simulink model "Test_FourMotor_PID_simcape_motor"  (R2025a)
settings: Solver=FixedStepAuto  StartTime=0.0  StopTime=2  FixedStep=50e-5  RelTol=1e-3
values from neighbouring files (symbols this model uses):
  Ki_id = 710.3004    [EMRAX348_DQData.m]    (also in Evolito_D500_DQData.m = 281.669634183)
  Ki_iq = 1.0615e3    (= 1061.5)    [EMRAX348_DQData.m]    (also in Evolito_D500_DQData.m = 420.937840785)
  Kp_id = 0.8779    [EMRAX348_DQData.m]    (also in Evolito_D500_DQData.m = 0.144107025607)
  Kp_iq = 1.0744    [EMRAX348_DQData.m]    (also in Evolito_D500_DQData.m = 0.144418307682)
  Ld = 52e-6    (= 5.2e-05)    [EMRAX348_DQData.m]    (also in Evolito_D500_DQData.m = 4e-05; pmsm_batt_testbench_data.m = 4e-05)
  Lq = 52e-6    (= 5.2e-05)    [EMRAX348_DQData.m]    (also in Evolito_D500_DQData.m = 4e-05; pmsm_batt_testbench_data.m = 4e-05)
  p = 10    [EMRAX348_DQData.m]    (also in Evolito_D500_DQData.m; pmsm_batt_testbench_data.m)
  psim = 0.06249    [EMRAX348_DQData.m]    (also in Evolito_D500_DQData.m = 0.045; pmsm_batt_testbench_data.m = 0.045)
undefined symbols (not defined in the file or in its folder): Limit, motorctrl, RPM
libraries: fl_lib x101, nesl_utility x37, eeDiscretePi x8, slpidlib x7, eeDqVoltageLimiter x4, eePmsmCurrentReferenceGen x4, eePmsmTorqueEstimator x4, ee_lib x4, batteryecm_lib x2, HEV_Battery_Lib x1, spspowerguiLib x1
(part 3 of 3)

== system Test_FourMotor_PID_simcape_motor/Detailed/Electric Drive/Sensor ==
  Filter A : TransferFcn  Denominator=[1e-4 1]
  Filter w : TransferFcn  Denominator=[1e-4 1]
  MRRef : fl_lib/Mechanical/Rotational Elements/Mechanical Rotational Reference
  Motion Sensor : fl_lib/Mechanical/Mechanical Sensors/Ideal Rotational Motion Sensor  reference=foundation.enum.MeasurementReference.difference  acceleration_port=false  velocity_port=true  position_port=true  wrap_angle=simscape.enum.onoff.off  offset=0 deg
  PS-Simulink Converter1 : nesl_utility/PS-Simulink Converter  PhysicalDomain=network_engine_domain  SubClassName=ps_output  LeftPortType=input  RightPortType=output  PseudoPeriodic=off  Frequencies=[]  VectorFormat=1-D array  Unit=rad/s  AffineConversion=off
  PS-Simulink Converter2 : nesl_utility/PS-Simulink Converter  PhysicalDomain=network_engine_domain  SubClassName=ps_output  LeftPortType=input  RightPortType=output  PseudoPeriodic=off  Frequencies=[]  VectorFormat=1-D array  Unit=rad  AffineConversion=off
  R : PMIOPort  Side=Left
  C : PMIOPort  Port=2  Side=Right
  w : Outport  VectorParamsAs1DForOutWhenUnconnected=off
  A : Outport  Port=2  VectorParamsAs1DForOutWhenUnconnected=off
  wires:
  PS-Simulink Converter1/1 -> Filter w/1
  PS-Simulink Converter2/1 -> Filter A/1
  Filter A/1 -> A/1
  Filter w/1 -> w/1
  connections:
  Motion Sensor/RConn2 -- PS-Simulink Converter1/LConn1
  Motion Sensor/RConn1 -- MRRef/LConn1
  C/RConn1 -- R/RConn1 -- Motion Sensor/LConn1
  Motion Sensor/RConn3 -- PS-Simulink Converter2/LConn1

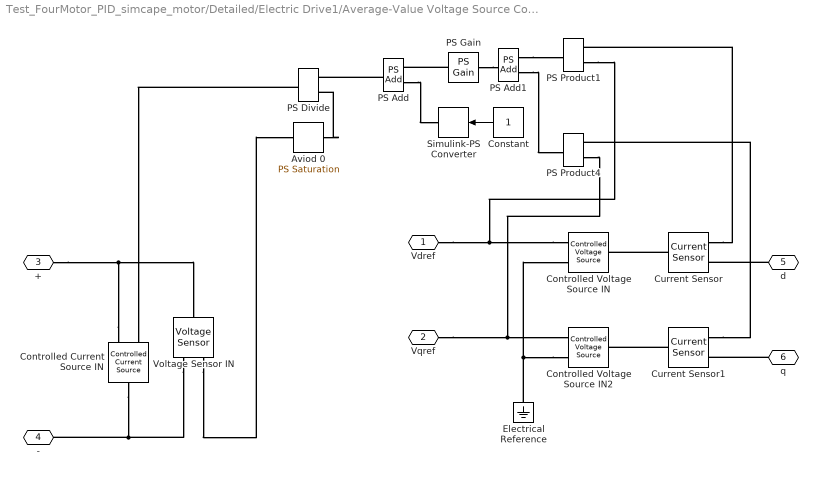
== system Test_FourMotor_PID_simcape_motor/Detailed/Electric Drive1/Average-Value Voltage Source Converter dq0 ==
  Aviod 0 : fl_lib/Physical Signals/Nonlinear Operators/PS Saturation  upper_limit=inf V  lower_limit=1e-6 V  ZeroCross=true
  Constant : Constant  SampleTime=0
  Controlled Current Source IN : fl_lib/Electrical/Electrical Sources/Controlled Current Source
  Controlled Voltage Source IN : fl_lib/Electrical/Electrical Sources/Controlled Voltage Source
  Controlled Voltage Source IN2 : fl_lib/Electrical/Electrical Sources/Controlled Voltage Source
  Current Sensor : fl_lib/Electrical/Electrical Sensors/Current Sensor
  Current Sensor1 : fl_lib/Electrical/Electrical Sensors/Current Sensor
  Electrical Reference : fl_lib/Electrical/Electrical Elements/Electrical Reference
  PS Add : fl_lib/Physical Signals/Functions/PS Add
  PS Add1 : fl_lib/Physical Signals/Functions/PS Add
  PS Divide : fl_lib/Physical Signals/Functions/PS Divide
  PS Gain : fl_lib/Physical Signals/Functions/PS Gain  gain=3/2
  PS Product1 : fl_lib/Physical Signals/Functions/PS Product
  PS Product4 : fl_lib/Physical Signals/Functions/PS Product
  Simulink-PS Converter : nesl_utility/Simulink-PS Converter  PhysicalDomain=network_engine_domain  SubClassName=ps_input  LeftPortType=input  RightPortType=output  PseudoPeriodic=off  Frequencies=[]  NoiseDistribution=none  NoiseParameters=[]  Unit=W  AffineConversion=off  FilteringAndDerivatives=provide  SimscapeFilterOrder=1  InputFilterTimeConstant=0.001  UdotUserProvided=0
  Voltage Sensor IN : fl_lib/Electrical/Electrical Sensors/Voltage Sensor
  Vdref : PMIOPort  Side=Left
  Vqref : PMIOPort  Port=2  Side=Left
  + : PMIOPort  Port=3  Side=Left
  - : PMIOPort  Port=4  Side=Left
  d : PMIOPort  Port=5  Side=Right
  q : PMIOPort  Port=6  Side=Right
  wires:
  Constant/1 -> Simulink-PS Converter/1
  connections:
  Controlled Current Source IN/RConn2 -- Voltage Sensor IN/LConn1 -- +/RConn1
  -/RConn1 -- Voltage Sensor IN/RConn2 -- Controlled Current Source IN/LConn1
  Controlled Voltage Source IN2/RConn2 -- Electrical Reference/LConn1 -- Controlled Voltage Source IN/RConn2
  Current Sensor1/LConn1 -- Controlled Voltage Source IN2/LConn1
  Current Sensor/LConn1 -- Controlled Voltage Source IN/LConn1
  Voltage Sensor IN/RConn1 -- Aviod 0/LConn1
  Controlled Voltage Source IN/RConn1 -- Vdref/RConn1 -- PS Product1/LConn2
  Vqref/RConn1 -- Controlled Voltage Source IN2/RConn1 -- PS Product4/LConn2
  PS Add1/LConn1 -- PS Product1/RConn1
  PS Add1/LConn2 -- PS Product4/RConn1
  Aviod 0/RConn1 -- PS Divide/LConn2
  PS Divide/RConn1 -- Controlled Current Source IN/RConn1
  PS Add/RConn1 -- PS Divide/LConn1
  PS Add/LConn2 -- Simulink-PS Converter/RConn1
  d/RConn1 -- Current Sensor/RConn2
  q/RConn1 -- Current Sensor1/RConn2
  Current Sensor/RConn1 -- PS Product1/LConn1
  Current Sensor1/RConn1 -- PS Product4/LConn1
  PS Gain/LConn1 -- PS Add1/RConn1
  PS Gain/RConn1 -- PS Add/LConn1

== system Test_FourMotor_PID_simcape_motor/Detailed/Electric Drive1/Meas I ==
  Current Sensor d : fl_lib/Electrical/Electrical Sensors/Current Sensor
  Current Sensor q : fl_lib/Electrical/Electrical Sensors/Current Sensor
  Filter id : TransferFcn  Denominator=[1e-4 1]
  Filter iq : TransferFcn  Denominator=[1e-4 1]
  Mux : Mux  Inputs=2
  PS-Simulink Converter : nesl_utility/PS-Simulink Converter  PhysicalDomain=network_engine_domain  SubClassName=ps_output  LeftPortType=input  RightPortType=output  PseudoPeriodic=off  Frequencies=[]  VectorFormat=1-D array  Unit=A  AffineConversion=off
  PS-Simulink Converter1 : nesl_utility/PS-Simulink Converter  PhysicalDomain=network_engine_domain  SubClassName=ps_output  LeftPortType=input  RightPortType=output  PseudoPeriodic=off  Frequencies=[]  VectorFormat=1-D array  Unit=A  AffineConversion=off
  d1 : PMIOPort  Side=Left
  q1 : PMIOPort  Port=2  Side=Left
  d2 : PMIOPort  Port=3  Side=Right
  q2 : PMIOPort  Port=4  Side=Right
  idq : Outport  VectorParamsAs1DForOutWhenUnconnected=off
  wires:
  PS-Simulink Converter1/1 -> Filter iq/1
  PS-Simulink Converter/1 -> Filter id/1
  Mux/1 -> idq/1
  Filter id/1 -> Mux/1
  Filter iq/1 -> Mux/2
  connections:
  d1/RConn1 -- Current Sensor d/LConn1
  Current Sensor q/LConn1 -- q1/RConn1
  Current Sensor d/RConn2 -- d2/RConn1
  q2/RConn1 -- Current Sensor q/RConn2
  PS-Simulink Converter/LConn1 -- Current Sensor d/RConn1
  PS-Simulink Converter1/LConn1 -- Current Sensor q/RConn1

== system Test_FourMotor_PID_simcape_motor/Detailed/Electric Drive1/Meas V ==
  PS-Simulink Converter4 : nesl_utility/PS-Simulink Converter  PhysicalDomain=network_engine_domain  SubClassName=ps_output  LeftPortType=input  RightPortType=output  PseudoPeriodic=off  Frequencies=[]  VectorFormat=1-D array  Unit=V  AffineConversion=off
  Voltage Sensor : fl_lib/Electrical/Electrical Sensors/Voltage Sensor
  - : PMIOPort  Side=Right
  + : PMIOPort  Port=2  Side=Left
  Vdc : Outport  VectorParamsAs1DForOutWhenUnconnected=off
  wires:
  PS-Simulink Converter4/1 -> Vdc/1
  connections:
  PS-Simulink Converter4/LConn1 -- Voltage Sensor/RConn1
  Voltage Sensor/LConn1 -- +/RConn1
  Voltage Sensor/RConn2 -- -/RConn1

== system Test_FourMotor_PID_simcape_motor/Detailed/Electric Drive1/Sensor ==
  Filter A : TransferFcn  Denominator=[1e-4 1]
  Filter w : TransferFcn  Denominator=[1e-4 1]
  MRRef : fl_lib/Mechanical/Rotational Elements/Mechanical Rotational Reference
  Motion Sensor : fl_lib/Mechanical/Mechanical Sensors/Ideal Rotational Motion Sensor  reference=foundation.enum.MeasurementReference.difference  acceleration_port=false  velocity_port=true  position_port=true  wrap_angle=simscape.enum.onoff.off  offset=0 deg
  PS-Simulink Converter1 : nesl_utility/PS-Simulink Converter  PhysicalDomain=network_engine_domain  SubClassName=ps_output  LeftPortType=input  RightPortType=output  PseudoPeriodic=off  Frequencies=[]  VectorFormat=1-D array  Unit=rad/s  AffineConversion=off
  PS-Simulink Converter2 : nesl_utility/PS-Simulink Converter  PhysicalDomain=network_engine_domain  SubClassName=ps_output  LeftPortType=input  RightPortType=output  PseudoPeriodic=off  Frequencies=[]  VectorFormat=1-D array  Unit=rad  AffineConversion=off
  R : PMIOPort  Side=Left
  C : PMIOPort  Port=2  Side=Right
  w : Outport  VectorParamsAs1DForOutWhenUnconnected=off
  A : Outport  Port=2  VectorParamsAs1DForOutWhenUnconnected=off
  wires:
  PS-Simulink Converter1/1 -> Filter w/1
  PS-Simulink Converter2/1 -> Filter A/1
  Filter A/1 -> A/1
  Filter w/1 -> w/1
  connections:
  Motion Sensor/RConn2 -- PS-Simulink Converter1/LConn1
  Motion Sensor/RConn1 -- MRRef/LConn1
  C/RConn1 -- R/RConn1 -- Motion Sensor/LConn1
  Motion Sensor/RConn3 -- PS-Simulink Converter2/LConn1

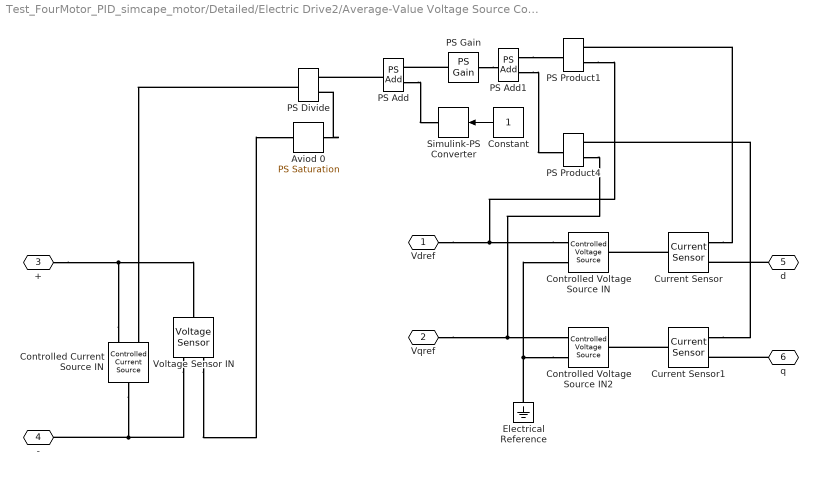
== system Test_FourMotor_PID_simcape_motor/Detailed/Electric Drive2/Average-Value Voltage Source Converter dq0 ==
  Aviod 0 : fl_lib/Physical Signals/Nonlinear Operators/PS Saturation  upper_limit=inf V  lower_limit=1e-6 V  ZeroCross=true
  Constant : Constant  SampleTime=0
  Controlled Current Source IN : fl_lib/Electrical/Electrical Sources/Controlled Current Source
  Controlled Voltage Source IN : fl_lib/Electrical/Electrical Sources/Controlled Voltage Source
  Controlled Voltage Source IN2 : fl_lib/Electrical/Electrical Sources/Controlled Voltage Source
  Current Sensor : fl_lib/Electrical/Electrical Sensors/Current Sensor
  Current Sensor1 : fl_lib/Electrical/Electrical Sensors/Current Sensor
  Electrical Reference : fl_lib/Electrical/Electrical Elements/Electrical Reference
  PS Add : fl_lib/Physical Signals/Functions/PS Add
  PS Add1 : fl_lib/Physical Signals/Functions/PS Add
  PS Divide : fl_lib/Physical Signals/Functions/PS Divide
  PS Gain : fl_lib/Physical Signals/Functions/PS Gain  gain=3/2
  PS Product1 : fl_lib/Physical Signals/Functions/PS Product
  PS Product4 : fl_lib/Physical Signals/Functions/PS Product
  Simulink-PS Converter : nesl_utility/Simulink-PS Converter  PhysicalDomain=network_engine_domain  SubClassName=ps_input  LeftPortType=input  RightPortType=output  PseudoPeriodic=off  Frequencies=[]  NoiseDistribution=none  NoiseParameters=[]  Unit=W  AffineConversion=off  FilteringAndDerivatives=provide  SimscapeFilterOrder=1  InputFilterTimeConstant=0.001  UdotUserProvided=0
  Voltage Sensor IN : fl_lib/Electrical/Electrical Sensors/Voltage Sensor
  Vdref : PMIOPort  Side=Left
  Vqref : PMIOPort  Port=2  Side=Left
  + : PMIOPort  Port=3  Side=Left
  - : PMIOPort  Port=4  Side=Left
  d : PMIOPort  Port=5  Side=Right
  q : PMIOPort  Port=6  Side=Right
  wires:
  Constant/1 -> Simulink-PS Converter/1
  connections:
  Controlled Current Source IN/RConn2 -- Voltage Sensor IN/LConn1 -- +/RConn1
  -/RConn1 -- Voltage Sensor IN/RConn2 -- Controlled Current Source IN/LConn1
  Controlled Voltage Source IN2/RConn2 -- Electrical Reference/LConn1 -- Controlled Voltage Source IN/RConn2
  Current Sensor1/LConn1 -- Controlled Voltage Source IN2/LConn1
  Current Sensor/LConn1 -- Controlled Voltage Source IN/LConn1
  Voltage Sensor IN/RConn1 -- Aviod 0/LConn1
  Controlled Voltage Source IN/RConn1 -- Vdref/RConn1 -- PS Product1/LConn2
  Vqref/RConn1 -- Controlled Voltage Source IN2/RConn1 -- PS Product4/LConn2
  PS Add1/LConn1 -- PS Product1/RConn1
  PS Add1/LConn2 -- PS Product4/RConn1
  Aviod 0/RConn1 -- PS Divide/LConn2
  PS Divide/RConn1 -- Controlled Current Source IN/RConn1
  PS Add/RConn1 -- PS Divide/LConn1
  PS Add/LConn2 -- Simulink-PS Converter/RConn1
  d/RConn1 -- Current Sensor/RConn2
  q/RConn1 -- Current Sensor1/RConn2
  Current Sensor/RConn1 -- PS Product1/LConn1
  Current Sensor1/RConn1 -- PS Product4/LConn1
  PS Gain/LConn1 -- PS Add1/RConn1
  PS Gain/RConn1 -- PS Add/LConn1

== system Test_FourMotor_PID_simcape_motor/Detailed/Electric Drive2/Meas I ==
  Current Sensor d : fl_lib/Electrical/Electrical Sensors/Current Sensor
  Current Sensor q : fl_lib/Electrical/Electrical Sensors/Current Sensor
  Filter id : TransferFcn  Denominator=[1e-4 1]
  Filter iq : TransferFcn  Denominator=[1e-4 1]
  Mux : Mux  Inputs=2
  PS-Simulink Converter : nesl_utility/PS-Simulink Converter  PhysicalDomain=network_engine_domain  SubClassName=ps_output  LeftPortType=input  RightPortType=output  PseudoPeriodic=off  Frequencies=[]  VectorFormat=1-D array  Unit=A  AffineConversion=off
  PS-Simulink Converter1 : nesl_utility/PS-Simulink Converter  PhysicalDomain=network_engine_domain  SubClassName=ps_output  LeftPortType=input  RightPortType=output  PseudoPeriodic=off  Frequencies=[]  VectorFormat=1-D array  Unit=A  AffineConversion=off
  d1 : PMIOPort  Side=Left
  q1 : PMIOPort  Port=2  Side=Left
  d2 : PMIOPort  Port=3  Side=Right
  q2 : PMIOPort  Port=4  Side=Right
  idq : Outport  VectorParamsAs1DForOutWhenUnconnected=off
  wires:
  PS-Simulink Converter1/1 -> Filter iq/1
  PS-Simulink Converter/1 -> Filter id/1
  Mux/1 -> idq/1
  Filter id/1 -> Mux/1
  Filter iq/1 -> Mux/2
  connections:
  d1/RConn1 -- Current Sensor d/LConn1
  Current Sensor q/LConn1 -- q1/RConn1
  Current Sensor d/RConn2 -- d2/RConn1
  q2/RConn1 -- Current Sensor q/RConn2
  PS-Simulink Converter/LConn1 -- Current Sensor d/RConn1
  PS-Simulink Converter1/LConn1 -- Current Sensor q/RConn1

== system Test_FourMotor_PID_simcape_motor/Detailed/Electric Drive2/Meas V ==
  PS-Simulink Converter4 : nesl_utility/PS-Simulink Converter  PhysicalDomain=network_engine_domain  SubClassName=ps_output  LeftPortType=input  RightPortType=output  PseudoPeriodic=off  Frequencies=[]  VectorFormat=1-D array  Unit=V  AffineConversion=off
  Voltage Sensor : fl_lib/Electrical/Electrical Sensors/Voltage Sensor
  - : PMIOPort  Side=Right
  + : PMIOPort  Port=2  Side=Left
  Vdc : Outport  VectorParamsAs1DForOutWhenUnconnected=off
  wires:
  PS-Simulink Converter4/1 -> Vdc/1
  connections:
  PS-Simulink Converter4/LConn1 -- Voltage Sensor/RConn1
  Voltage Sensor/LConn1 -- +/RConn1
  Voltage Sensor/RConn2 -- -/RConn1

== system Test_FourMotor_PID_simcape_motor/Detailed/Electric Drive2/Sensor ==
  Filter A : TransferFcn  Denominator=[1e-4 1]
  Filter w : TransferFcn  Denominator=[1e-4 1]
  MRRef : fl_lib/Mechanical/Rotational Elements/Mechanical Rotational Reference
  Motion Sensor : fl_lib/Mechanical/Mechanical Sensors/Ideal Rotational Motion Sensor  reference=foundation.enum.MeasurementReference.difference  acceleration_port=false  velocity_port=true  position_port=true  wrap_angle=simscape.enum.onoff.off  offset=0 deg
  PS-Simulink Converter1 : nesl_utility/PS-Simulink Converter  PhysicalDomain=network_engine_domain  SubClassName=ps_output  LeftPortType=input  RightPortType=output  PseudoPeriodic=off  Frequencies=[]  VectorFormat=1-D array  Unit=rad/s  AffineConversion=off
  PS-Simulink Converter2 : nesl_utility/PS-Simulink Converter  PhysicalDomain=network_engine_domain  SubClassName=ps_output  LeftPortType=input  RightPortType=output  PseudoPeriodic=off  Frequencies=[]  VectorFormat=1-D array  Unit=rad  AffineConversion=off
  R : PMIOPort  Side=Left
  C : PMIOPort  Port=2  Side=Right
  w : Outport  VectorParamsAs1DForOutWhenUnconnected=off
  A : Outport  Port=2  VectorParamsAs1DForOutWhenUnconnected=off
  wires:
  PS-Simulink Converter1/1 -> Filter w/1
  PS-Simulink Converter2/1 -> Filter A/1
  Filter A/1 -> A/1
  Filter w/1 -> w/1
  connections:
  Motion Sensor/RConn2 -- PS-Simulink Converter1/LConn1
  Motion Sensor/RConn1 -- MRRef/LConn1
  C/RConn1 -- R/RConn1 -- Motion Sensor/LConn1
  Motion Sensor/RConn3 -- PS-Simulink Converter2/LConn1

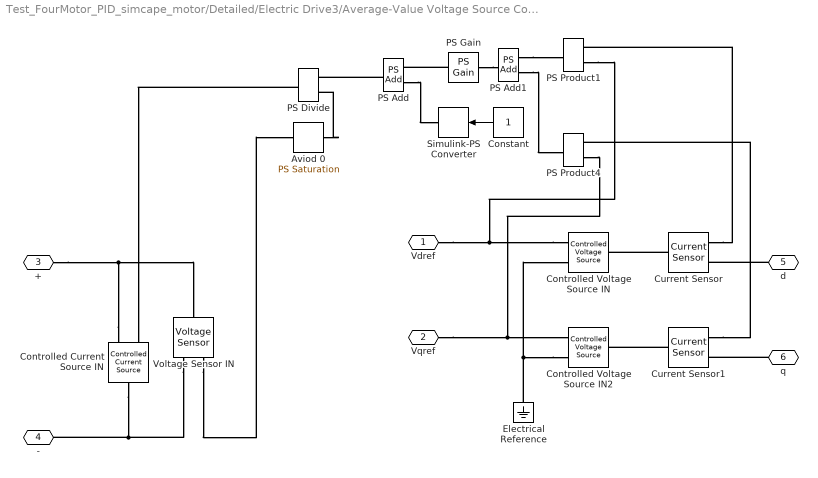
== system Test_FourMotor_PID_simcape_motor/Detailed/Electric Drive3/Average-Value Voltage Source Converter dq0 ==
  Aviod 0 : fl_lib/Physical Signals/Nonlinear Operators/PS Saturation  upper_limit=inf V  lower_limit=1e-6 V  ZeroCross=true
  Constant : Constant  SampleTime=0
  Controlled Current Source IN : fl_lib/Electrical/Electrical Sources/Controlled Current Source
  Controlled Voltage Source IN : fl_lib/Electrical/Electrical Sources/Controlled Voltage Source
  Controlled Voltage Source IN2 : fl_lib/Electrical/Electrical Sources/Controlled Voltage Source
  Current Sensor : fl_lib/Electrical/Electrical Sensors/Current Sensor
  Current Sensor1 : fl_lib/Electrical/Electrical Sensors/Current Sensor
  Electrical Reference : fl_lib/Electrical/Electrical Elements/Electrical Reference
  PS Add : fl_lib/Physical Signals/Functions/PS Add
  PS Add1 : fl_lib/Physical Signals/Functions/PS Add
  PS Divide : fl_lib/Physical Signals/Functions/PS Divide
  PS Gain : fl_lib/Physical Signals/Functions/PS Gain  gain=3/2
  PS Product1 : fl_lib/Physical Signals/Functions/PS Product
  PS Product4 : fl_lib/Physical Signals/Functions/PS Product
  Simulink-PS Converter : nesl_utility/Simulink-PS Converter  PhysicalDomain=network_engine_domain  SubClassName=ps_input  LeftPortType=input  RightPortType=output  PseudoPeriodic=off  Frequencies=[]  NoiseDistribution=none  NoiseParameters=[]  Unit=W  AffineConversion=off  FilteringAndDerivatives=provide  SimscapeFilterOrder=1  InputFilterTimeConstant=0.001  UdotUserProvided=0
  Voltage Sensor IN : fl_lib/Electrical/Electrical Sensors/Voltage Sensor
  Vdref : PMIOPort  Side=Left
  Vqref : PMIOPort  Port=2  Side=Left
  + : PMIOPort  Port=3  Side=Left
  - : PMIOPort  Port=4  Side=Left
  d : PMIOPort  Port=5  Side=Right
  q : PMIOPort  Port=6  Side=Right
  wires:
  Constant/1 -> Simulink-PS Converter/1
  connections:
  Controlled Current Source IN/RConn2 -- Voltage Sensor IN/LConn1 -- +/RConn1
  -/RConn1 -- Voltage Sensor IN/RConn2 -- Controlled Current Source IN/LConn1
  Controlled Voltage Source IN2/RConn2 -- Electrical Reference/LConn1 -- Controlled Voltage Source IN/RConn2
  Current Sensor1/LConn1 -- Controlled Voltage Source IN2/LConn1
  Current Sensor/LConn1 -- Controlled Voltage Source IN/LConn1
  Voltage Sensor IN/RConn1 -- Aviod 0/LConn1
  Controlled Voltage Source IN/RConn1 -- Vdref/RConn1 -- PS Product1/LConn2
  Vqref/RConn1 -- Controlled Voltage Source IN2/RConn1 -- PS Product4/LConn2
  PS Add1/LConn1 -- PS Product1/RConn1
  PS Add1/LConn2 -- PS Product4/RConn1
  Aviod 0/RConn1 -- PS Divide/LConn2
  PS Divide/RConn1 -- Controlled Current Source IN/RConn1
  PS Add/RConn1 -- PS Divide/LConn1
  PS Add/LConn2 -- Simulink-PS Converter/RConn1
  d/RConn1 -- Current Sensor/RConn2
  q/RConn1 -- Current Sensor1/RConn2
  Current Sensor/RConn1 -- PS Product1/LConn1
  Current Sensor1/RConn1 -- PS Product4/LConn1
  PS Gain/LConn1 -- PS Add1/RConn1
  PS Gain/RConn1 -- PS Add/LConn1

== system Test_FourMotor_PID_simcape_motor/Detailed/Electric Drive3/Meas I ==
  Current Sensor d : fl_lib/Electrical/Electrical Sensors/Current Sensor
  Current Sensor q : fl_lib/Electrical/Electrical Sensors/Current Sensor
  Filter id : TransferFcn  Denominator=[1e-4 1]
  Filter iq : TransferFcn  Denominator=[1e-4 1]
  Mux : Mux  Inputs=2
  PS-Simulink Converter : nesl_utility/PS-Simulink Converter  PhysicalDomain=network_engine_domain  SubClassName=ps_output  LeftPortType=input  RightPortType=output  PseudoPeriodic=off  Frequencies=[]  VectorFormat=1-D array  Unit=A  AffineConversion=off
  PS-Simulink Converter1 : nesl_utility/PS-Simulink Converter  PhysicalDomain=network_engine_domain  SubClassName=ps_output  LeftPortType=input  RightPortType=output  PseudoPeriodic=off  Frequencies=[]  VectorFormat=1-D array  Unit=A  AffineConversion=off
  d1 : PMIOPort  Side=Left
  q1 : PMIOPort  Port=2  Side=Left
  d2 : PMIOPort  Port=3  Side=Right
  q2 : PMIOPort  Port=4  Side=Right
  idq : Outport  VectorParamsAs1DForOutWhenUnconnected=off
  wires:
  PS-Simulink Converter1/1 -> Filter iq/1
  PS-Simulink Converter/1 -> Filter id/1
  Mux/1 -> idq/1
  Filter id/1 -> Mux/1
  Filter iq/1 -> Mux/2
  connections:
  d1/RConn1 -- Current Sensor d/LConn1
  Current Sensor q/LConn1 -- q1/RConn1
  Current Sensor d/RConn2 -- d2/RConn1
  q2/RConn1 -- Current Sensor q/RConn2
  PS-Simulink Converter/LConn1 -- Current Sensor d/RConn1
  PS-Simulink Converter1/LConn1 -- Current Sensor q/RConn1

== system Test_FourMotor_PID_simcape_motor/Detailed/Electric Drive3/Meas V ==
  PS-Simulink Converter4 : nesl_utility/PS-Simulink Converter  PhysicalDomain=network_engine_domain  SubClassName=ps_output  LeftPortType=input  RightPortType=output  PseudoPeriodic=off  Frequencies=[]  VectorFormat=1-D array  Unit=V  AffineConversion=off
  Voltage Sensor : fl_lib/Electrical/Electrical Sensors/Voltage Sensor
  - : PMIOPort  Side=Right
  + : PMIOPort  Port=2  Side=Left
  Vdc : Outport  VectorParamsAs1DForOutWhenUnconnected=off
  wires:
  PS-Simulink Converter4/1 -> Vdc/1
  connections:
  PS-Simulink Converter4/LConn1 -- Voltage Sensor/RConn1
  Voltage Sensor/LConn1 -- +/RConn1
  Voltage Sensor/RConn2 -- -/RConn1

== system Test_FourMotor_PID_simcape_motor/Detailed/Electric Drive3/Sensor ==
  Filter A : TransferFcn  Denominator=[1e-4 1]
  Filter w : TransferFcn  Denominator=[1e-4 1]
  MRRef : fl_lib/Mechanical/Rotational Elements/Mechanical Rotational Reference
  Motion Sensor : fl_lib/Mechanical/Mechanical Sensors/Ideal Rotational Motion Sensor  reference=foundation.enum.MeasurementReference.difference  acceleration_port=false  velocity_port=true  position_port=true  wrap_angle=simscape.enum.onoff.off  offset=0 deg
  PS-Simulink Converter1 : nesl_utility/PS-Simulink Converter  PhysicalDomain=network_engine_domain  SubClassName=ps_output  LeftPortType=input  RightPortType=output  PseudoPeriodic=off  Frequencies=[]  VectorFormat=1-D array  Unit=rad/s  AffineConversion=off
  PS-Simulink Converter2 : nesl_utility/PS-Simulink Converter  PhysicalDomain=network_engine_domain  SubClassName=ps_output  LeftPortType=input  RightPortType=output  PseudoPeriodic=off  Frequencies=[]  VectorFormat=1-D array  Unit=rad  AffineConversion=off
  R : PMIOPort  Side=Left
  C : PMIOPort  Port=2  Side=Right
  w : Outport  VectorParamsAs1DForOutWhenUnconnected=off
  A : Outport  Port=2  VectorParamsAs1DForOutWhenUnconnected=off
  wires:
  PS-Simulink Converter1/1 -> Filter w/1
  PS-Simulink Converter2/1 -> Filter A/1
  Filter A/1 -> A/1
  Filter w/1 -> w/1
  connections:
  Motion Sensor/RConn2 -- PS-Simulink Converter1/LConn1
  Motion Sensor/RConn1 -- MRRef/LConn1
  C/RConn1 -- R/RConn1 -- Motion Sensor/LConn1
  Motion Sensor/RConn3 -- PS-Simulink Converter2/LConn1

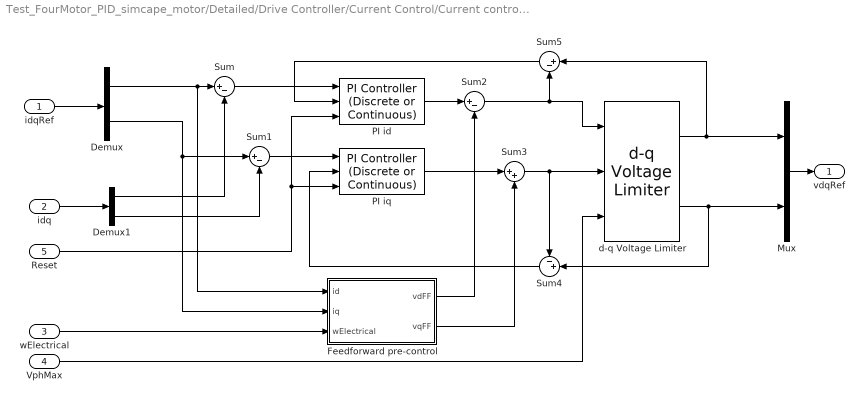
== system Test_FourMotor_PID_simcape_motor/Detailed/Drive Controller/Current Control/Current controller ==
  idqRef : Inport
  idq : Inport  Port=2
  wElectrical : Inport  Port=3
  VphMax : Inport  Port=4
  Reset : Inport  Port=5
  Demux : Demux  Outputs=2
  Demux1 : Demux  Outputs=2
  Feedforward pre-control : Subsystem
  Mux : Mux  Inputs=2
  PI id : eeDiscretePi/PI Controller (Discrete or Continuous)  Kp=Kp_id  Ki=Ki_id  Kaw=1  x0=0  Ts=0
  PI iq : eeDiscretePi/PI Controller (Discrete or Continuous)  Kp=Kp_iq  Ki=Ki_iq  Kaw=1  x0=0  Ts=0
  Sum{,1..2,5} (4 alike) : Sum  Inputs=|+-
  Sum3 : Sum  Inputs=|++
  Sum4 : Sum  Inputs=-+|
  d-q Voltage Limiter : eeDqVoltageLimiter/d-q Voltage Limiter  AxisPrio=Q-axis  Ts=0
  vdqRef : Outport  VectorParamsAs1DForOutWhenUnconnected=off
  wires:
  Demux1/1 -> Sum/2
  idq/1 -> Demux1/1
  Demux/2 -> Feedforward pre-control/2(iq), Sum1/1
  Reset/1 -> PI id/3, PI iq/3
  Sum3/1 -> Sum4/1, d-q Voltage Limiter/2
  Sum4/1 -> PI iq/2
  VphMax/1 -> d-q Voltage Limiter/3
  Mux/1 -> vdqRef/1
  Feedforward pre-control/2(vqFF) -> Sum3/2
  wElectrical/1 -> Feedforward pre-control/3(wElectrical)
  idqRef/1 -> Demux/1
  Sum/1 -> PI id/1
  PI id/1 -> Sum2/1
  Sum5/1 -> PI id/2
  PI iq/1 -> Sum3/1
  Feedforward pre-control/1(vdFF) -> Sum2/2
  Sum1/1 -> PI iq/1
  Demux/1 -> Sum/1, Feedforward pre-control/1(id)
  Demux1/2 -> Sum1/2
  Sum2/1 -> Sum5/2, d-q Voltage Limiter/1
  d-q Voltage Limiter/1 -> Mux/1, Sum5/1
  d-q Voltage Limiter/2 -> Mux/2, Sum4/2

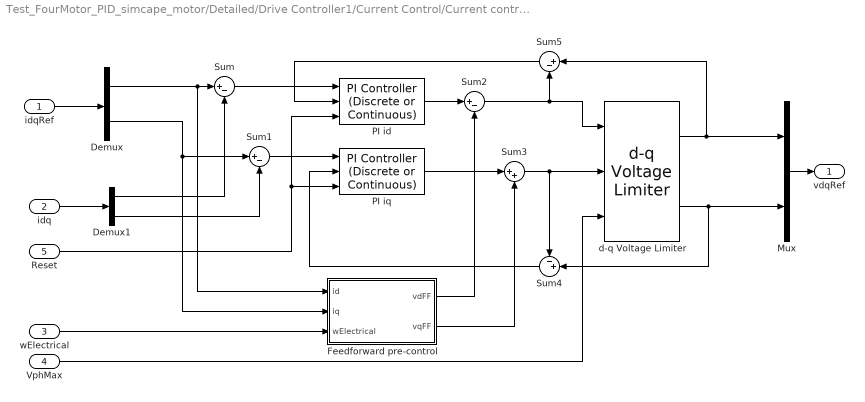
== system Test_FourMotor_PID_simcape_motor/Detailed/Drive Controller1/Current Control/Current controller ==
  idqRef : Inport
  idq : Inport  Port=2
  wElectrical : Inport  Port=3
  VphMax : Inport  Port=4
  Reset : Inport  Port=5
  Demux : Demux  Outputs=2
  Demux1 : Demux  Outputs=2
  Feedforward pre-control : Subsystem
  Mux : Mux  Inputs=2
  PI id : eeDiscretePi/PI Controller (Discrete or Continuous)  Kp=Kp_id  Ki=Ki_id  Kaw=1  x0=0  Ts=0
  PI iq : eeDiscretePi/PI Controller (Discrete or Continuous)  Kp=Kp_iq  Ki=Ki_iq  Kaw=1  x0=0  Ts=0
  Sum{,1..2,5} (4 alike) : Sum  Inputs=|+-
  Sum3 : Sum  Inputs=|++
  Sum4 : Sum  Inputs=-+|
  d-q Voltage Limiter : eeDqVoltageLimiter/d-q Voltage Limiter  AxisPrio=Q-axis  Ts=0
  vdqRef : Outport  VectorParamsAs1DForOutWhenUnconnected=off
  wires:
  Demux1/1 -> Sum/2
  idq/1 -> Demux1/1
  Demux/2 -> Feedforward pre-control/2(iq), Sum1/1
  Reset/1 -> PI id/3, PI iq/3
  Sum3/1 -> Sum4/1, d-q Voltage Limiter/2
  Sum4/1 -> PI iq/2
  VphMax/1 -> d-q Voltage Limiter/3
  Mux/1 -> vdqRef/1
  Feedforward pre-control/2(vqFF) -> Sum3/2
  wElectrical/1 -> Feedforward pre-control/3(wElectrical)
  idqRef/1 -> Demux/1
  Sum/1 -> PI id/1
  PI id/1 -> Sum2/1
  Sum5/1 -> PI id/2
  PI iq/1 -> Sum3/1
  Feedforward pre-control/1(vdFF) -> Sum2/2
  Sum1/1 -> PI iq/1
  Demux/1 -> Sum/1, Feedforward pre-control/1(id)
  Demux1/2 -> Sum1/2
  Sum2/1 -> Sum5/2, d-q Voltage Limiter/1
  d-q Voltage Limiter/1 -> Mux/1, Sum5/1
  d-q Voltage Limiter/2 -> Mux/2, Sum4/2

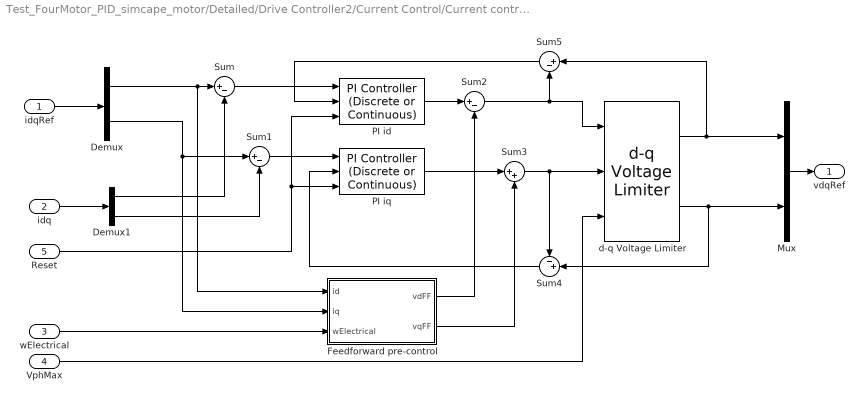
== system Test_FourMotor_PID_simcape_motor/Detailed/Drive Controller2/Current Control/Current controller ==
  idqRef : Inport
  idq : Inport  Port=2
  wElectrical : Inport  Port=3
  VphMax : Inport  Port=4
  Reset : Inport  Port=5
  Demux : Demux  Outputs=2
  Demux1 : Demux  Outputs=2
  Feedforward pre-control : Subsystem
  Mux : Mux  Inputs=2
  PI id : eeDiscretePi/PI Controller (Discrete or Continuous)  Kp=Kp_id  Ki=Ki_id  Kaw=1  x0=0  Ts=0
  PI iq : eeDiscretePi/PI Controller (Discrete or Continuous)  Kp=Kp_iq  Ki=Ki_iq  Kaw=1  x0=0  Ts=0
  Sum{,1..2,5} (4 alike) : Sum  Inputs=|+-
  Sum3 : Sum  Inputs=|++
  Sum4 : Sum  Inputs=-+|
  d-q Voltage Limiter : eeDqVoltageLimiter/d-q Voltage Limiter  AxisPrio=Q-axis  Ts=0
  vdqRef : Outport  VectorParamsAs1DForOutWhenUnconnected=off
  wires:
  Demux1/1 -> Sum/2
  idq/1 -> Demux1/1
  Demux/2 -> Feedforward pre-control/2(iq), Sum1/1
  Reset/1 -> PI id/3, PI iq/3
  Sum3/1 -> Sum4/1, d-q Voltage Limiter/2
  Sum4/1 -> PI iq/2
  VphMax/1 -> d-q Voltage Limiter/3
  Mux/1 -> vdqRef/1
  Feedforward pre-control/2(vqFF) -> Sum3/2
  wElectrical/1 -> Feedforward pre-control/3(wElectrical)
  idqRef/1 -> Demux/1
  Sum/1 -> PI id/1
  PI id/1 -> Sum2/1
  Sum5/1 -> PI id/2
  PI iq/1 -> Sum3/1
  Feedforward pre-control/1(vdFF) -> Sum2/2
  Sum1/1 -> PI iq/1
  Demux/1 -> Sum/1, Feedforward pre-control/1(id)
  Demux1/2 -> Sum1/2
  Sum2/1 -> Sum5/2, d-q Voltage Limiter/1
  d-q Voltage Limiter/1 -> Mux/1, Sum5/1
  d-q Voltage Limiter/2 -> Mux/2, Sum4/2

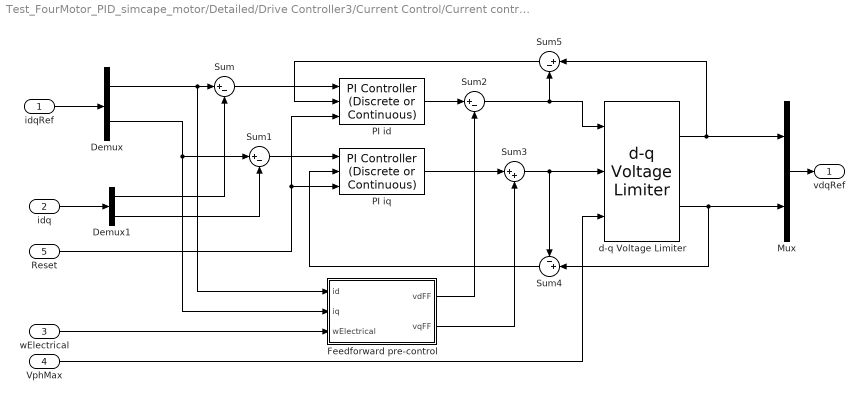
== system Test_FourMotor_PID_simcape_motor/Detailed/Drive Controller3/Current Control/Current controller ==
  idqRef : Inport
  idq : Inport  Port=2
  wElectrical : Inport  Port=3
  VphMax : Inport  Port=4
  Reset : Inport  Port=5
  Demux : Demux  Outputs=2
  Demux1 : Demux  Outputs=2
  Feedforward pre-control : Subsystem
  Mux : Mux  Inputs=2
  PI id : eeDiscretePi/PI Controller (Discrete or Continuous)  Kp=Kp_id  Ki=Ki_id  Kaw=1  x0=0  Ts=0
  PI iq : eeDiscretePi/PI Controller (Discrete or Continuous)  Kp=Kp_iq  Ki=Ki_iq  Kaw=1  x0=0  Ts=0
  Sum{,1..2,5} (4 alike) : Sum  Inputs=|+-
  Sum3 : Sum  Inputs=|++
  Sum4 : Sum  Inputs=-+|
  d-q Voltage Limiter : eeDqVoltageLimiter/d-q Voltage Limiter  AxisPrio=Q-axis  Ts=0
  vdqRef : Outport  VectorParamsAs1DForOutWhenUnconnected=off
  wires:
  Demux1/1 -> Sum/2
  idq/1 -> Demux1/1
  Demux/2 -> Feedforward pre-control/2(iq), Sum1/1
  Reset/1 -> PI id/3, PI iq/3
  Sum3/1 -> Sum4/1, d-q Voltage Limiter/2
  Sum4/1 -> PI iq/2
  VphMax/1 -> d-q Voltage Limiter/3
  Mux/1 -> vdqRef/1
  Feedforward pre-control/2(vqFF) -> Sum3/2
  wElectrical/1 -> Feedforward pre-control/3(wElectrical)
  idqRef/1 -> Demux/1
  Sum/1 -> PI id/1
  PI id/1 -> Sum2/1
  Sum5/1 -> PI id/2
  PI iq/1 -> Sum3/1
  Feedforward pre-control/1(vdFF) -> Sum2/2
  Sum1/1 -> PI iq/1
  Demux/1 -> Sum/1, Feedforward pre-control/1(id)
  Demux1/2 -> Sum1/2
  Sum2/1 -> Sum5/2, d-q Voltage Limiter/1
  d-q Voltage Limiter/1 -> Mux/1, Sum5/1
  d-q Voltage Limiter/2 -> Mux/2, Sum4/2

== system Test_FourMotor_PID_simcape_motor/Detailed/Drive Controller/Current Control/Current controller/Feedforward pre-control ==
  id : Inport
  iq : Inport  Port=2
  wElectrical : Inport  Port=3
  Constant1 : Constant  Value=Ld
  Constant2 : Constant  Value=Lq
  Constant3 : Constant  Value=psim
  Demux : Demux  Outputs=2
  Mux1 : Mux  Inputs=2
  Product2 : Product  Inputs=3
  Product3 : Product
  Product4 : Product  Inputs=3
  Sum1 : Sum
  vdFF : Outport  VectorParamsAs1DForOutWhenUnconnected=off
  vqFF : Outport  Port=2  VectorParamsAs1DForOutWhenUnconnected=off
  wires:
  Product2/1 -> Sum1/1
  wElectrical/1 -> Product2/3, Product4/3, Product3/2
  Product4/1 -> Mux1/1
  id/1 -> Product2/1
  iq/1 -> Product4/1
  Constant1/1 -> Product2/2
  Sum1/1 -> Mux1/2
  Constant3/1 -> Product3/1
  Demux/2 -> vqFF/1
  Demux/1 -> vdFF/1
  Mux1/1 -> Demux/1
  Constant2/1 -> Product4/2
  Product3/1 -> Sum1/2

== system Test_FourMotor_PID_simcape_motor/Detailed/Drive Controller1/Current Control/Current controller/Feedforward pre-control ==
  id : Inport
  iq : Inport  Port=2
  wElectrical : Inport  Port=3
  Constant1 : Constant  Value=Ld
  Constant2 : Constant  Value=Lq
  Constant3 : Constant  Value=psim
  Demux : Demux  Outputs=2
  Mux1 : Mux  Inputs=2
  Product2 : Product  Inputs=3
  Product3 : Product
  Product4 : Product  Inputs=3
  Sum1 : Sum
  vdFF : Outport  VectorParamsAs1DForOutWhenUnconnected=off
  vqFF : Outport  Port=2  VectorParamsAs1DForOutWhenUnconnected=off
  wires:
  Product2/1 -> Sum1/1
  wElectrical/1 -> Product2/3, Product4/3, Product3/2
  Product4/1 -> Mux1/1
  id/1 -> Product2/1
  iq/1 -> Product4/1
  Constant1/1 -> Product2/2
  Sum1/1 -> Mux1/2
  Constant3/1 -> Product3/1
  Demux/2 -> vqFF/1
  Demux/1 -> vdFF/1
  Mux1/1 -> Demux/1
  Constant2/1 -> Product4/2
  Product3/1 -> Sum1/2

== system Test_FourMotor_PID_simcape_motor/Detailed/Drive Controller2/Current Control/Current controller/Feedforward pre-control ==
  id : Inport
  iq : Inport  Port=2
  wElectrical : Inport  Port=3
  Constant1 : Constant  Value=Ld
  Constant2 : Constant  Value=Lq
  Constant3 : Constant  Value=psim
  Demux : Demux  Outputs=2
  Mux1 : Mux  Inputs=2
  Product2 : Product  Inputs=3
  Product3 : Product
  Product4 : Product  Inputs=3
  Sum1 : Sum
  vdFF : Outport  VectorParamsAs1DForOutWhenUnconnected=off
  vqFF : Outport  Port=2  VectorParamsAs1DForOutWhenUnconnected=off
  wires:
  Product2/1 -> Sum1/1
  wElectrical/1 -> Product2/3, Product4/3, Product3/2
  Product4/1 -> Mux1/1
  id/1 -> Product2/1
  iq/1 -> Product4/1
  Constant1/1 -> Product2/2
  Sum1/1 -> Mux1/2
  Constant3/1 -> Product3/1
  Demux/2 -> vqFF/1
  Demux/1 -> vdFF/1
  Mux1/1 -> Demux/1
  Constant2/1 -> Product4/2
  Product3/1 -> Sum1/2

== system Test_FourMotor_PID_simcape_motor/Detailed/Drive Controller3/Current Control/Current controller/Feedforward pre-control ==
  id : Inport
  iq : Inport  Port=2
  wElectrical : Inport  Port=3
  Constant1 : Constant  Value=Ld
  Constant2 : Constant  Value=Lq
  Constant3 : Constant  Value=psim
  Demux : Demux  Outputs=2
  Mux1 : Mux  Inputs=2
  Product2 : Product  Inputs=3
  Product3 : Product
  Product4 : Product  Inputs=3
  Sum1 : Sum
  vdFF : Outport  VectorParamsAs1DForOutWhenUnconnected=off
  vqFF : Outport  Port=2  VectorParamsAs1DForOutWhenUnconnected=off
  wires:
  Product2/1 -> Sum1/1
  wElectrical/1 -> Product2/3, Product4/3, Product3/2
  Product4/1 -> Mux1/1
  id/1 -> Product2/1
  iq/1 -> Product4/1
  Constant1/1 -> Product2/2
  Sum1/1 -> Mux1/2
  Constant3/1 -> Product3/1
  Demux/2 -> vqFF/1
  Demux/1 -> vdFF/1
  Mux1/1 -> Demux/1
  Constant2/1 -> Product4/2
  Product3/1 -> Sum1/2
